simulink model "Interface_Model"  (R2017b)
settings: Solver=FixedStepDiscrete  StartTime=0.0  StopTime=inf  RelTol=1e-3  EnableMultiTasking=on
InitFcn:
  | modelSettings
undefined symbols (not defined in the file or in its folder): F, RadioSampleRate
libraries: gm_combinedTxRx_ExternalMode_lib x3
settings Model: SimulationMode=external  Creator=tcollins  LastModifiedBy=tcollins
settings SolverCC: PositivePriorityOrder=on
settings OptimizationCC: BlockReduction=off  ConditionallyExecuteInputs=off  PassReuseOutputArgsAs=Individual arguments  MaxStackSize=64
settings DebuggingCC: AlgebraicLoopMsg=error  SingleTaskRateTransMsg=error  ParameterTunabilityLossMsg=error
settings HardwareCC: ProdBitPerPointer=32  ProdBitPerSizeT=32  ProdBitPerPtrDiffT=32  ProdLargestAtomicInteger=Long  ProdLargestAtomicFloat=Double  ProdWordSize=32  ProdLongLongMode=on  ProdHWDeviceType=ARM Compatible->ARM Cortex  TargetLargestAtomicInteger=Long  TargetLargestAtomicFloat=Double  TargetIntDivRoundTo=Zero  TargetEndianess=LittleEndian  TargetHWDeviceType=ARM Compatible->ARM Cortex
settings SFSimCC: MATLABDynamicMemAlloc=off
settings RTWCC: SystemTargetFile=ert.tlc  HardwareBoard=Xilinx Zynq Based Radio Board Target  TemplateMakefile=ert_default_tmf  GenerateReport=on  Toolchain=Xilinx Software Development Kit (SDK)  IncludeHyperlinkInReport=on  LaunchReport=on  GenerateTraceInfo=on  GenerateTraceReport=on  GenerateTraceReportSl=on  GenerateTraceReportSf=on  GenerateTraceReportEml=on
settings CodeAppCC: ForceParamTrailComments=on  IgnoreCustomStorageClasses=off  OperatorAnnotations=on  SimulinkDataObjDesc=on  SFDataObjDesc=on  InsertBlockDesc=on

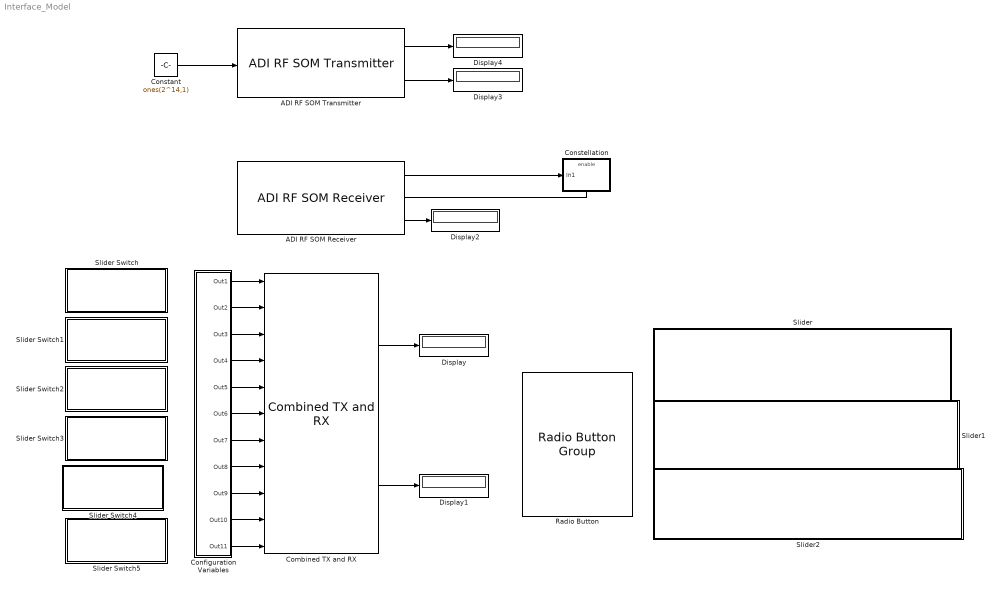
== system Interface_Model ==
  ADI RF SOM Receiver : gm_combinedTxRx_ExternalMode_lib/ADI RF SOM Receiver  IPAddress=192.168.3.2  CenterFrequencySource=Dialog  CenterFrequency=2400000000  GainSource=AGC Slow Attack  Gain=1  ChannelMapping=1  BasebandSampleRate=1e6  EnableBurstMode=off  NumFramesInBurst=20  OutputDataType=int16  SamplesPerFrame=2^14  LostSamplesOutputPort=on  RSSIOutputPort=off  DMATimeoutValue=1  blockMode=Codegen  SimulateUsing=Code generation  EnableQuadratureTracking=on  EnableRFDCTracking=on  EnableBasebandDCTracking=on  BypassUserLogic=off  ShowAdvancedProperties=on  ShowInternalProperties=off  subDeviceList=zynqReceiver  sdrExecutionMode=HW  dataUDPPort=-1  ctrlUDPPort=-1  SourceSelect=RF data  SourceConfiguration1=1023  FIRCoefficientSize=[ 128; 128 ]  FIRCoefficients=[ 55, -54, 42, -126, -123, -317, -399, -581, -646, -711, -634, -507, -263, -10, 255, 424, 492, 401, 201, -84, -352, -540, -566, -423, -126, 234, 562, 738, 701, 429, -5, -490, -866, -1007, -834, -372, 266, 891, 1301, 1334, 936, 178, -733, -1524, -1917, -1731, -944, 274, 1590, 2585, 2881, 2255, 741, -1344, -3435, -4850, -4942, -3285, 197, 5169, 10923, 16509, 20932, 23375, 23375, 20932, 16509, 10923, 5169, 197, -3285, -4942, -4850, -3435, -1344, 741, 2255, 2881, 2585, 1590, 274, -944, -1731, -1917, -1524, -733, 178, 936, 1334, 1301, 891, 266, -372, -834, -1007, -866, -490, -5, 429, 701, 738, 562, 234, -126, -423, -566, -540, -352, -84, 201, 401, 492, 424, 255, -10, -263, -507, -634, -711, -646, -581, -399, -317, -123, -126, 42, -54, 55; 190, -88, 329, -40, 239, -99, -24, -349, -377, -611, -573, -604, -395, -229, 66, 239, 394, 350, 227, -46, -300, -534, -593, -506, -221, 137, 512, 737, 765, 526, 103, -420, -852, -1069, -947, -512, 156, 841, 1341, 1450, 1100, 333, -638, -1531, -2028, -1922, -1152, 115, 1544, 2677, 3099, 2535, 997, -1205, -3479, -5095, -5345, -3750, -199, 4965, 11002, 16895, 21580, 24172, 24172, 21580, 16895, 11002, 4965, -199, -3750, -5345, -5095, -3479, -1205, 997, 2535, 3099, 2677, 1544, 115, -1152, -1922, -2028, -1531, -638, 333, 1100, 1450, 1341, 841, 156, -512, -947, -1069, -852, -420, 103, 526, 765, 737, 512, 137, -221, -506, -593, -534, -300, -46, 227, 350, 394, 239, 66, -229, -395, -604, -573, -611, -377, -349, -24, -99, 239, -40, 329, -88, 190 ]  FIRGain=[ 0; -12 ]  FIRDecimInterpFactor=[ 4; 4 ]  AnalogFilterCutoff=[ 3152524; 3161715 ]  FilterPathRates=[ 983040000, 122880000, 61440000, 30720000, 15360000, 3840000; 983040000, 122880000, 61440000, 30720000, 15360000, 3840000 ]  FilterDesignTypeForTx=DefaultFilterFromOther  FilterDesignTypeForRx=DefaultFilter  BISTLoopbackConfig=No Loopback  BISTPRBSMode=PRBS Disable  BISTToneMode=Tone Disable  BISTToneFrequency=F/32  BISTToneLevel=-6  BISTChannelMask=0  DataIsComplex=on
  ADI RF SOM Transmitter : gm_combinedTxRx_ExternalMode_lib/ADI RF SOM Transmitter  IPAddress=192.168.3.2  CenterFrequencySource=Dialog  CenterFrequency=2400000000  GainSource=Dialog  Gain=-10  ChannelMapping=1  BasebandSampleRate=1e6  EnableBurstMode=off  NumFramesInBurst=20  DMATimeoutValue=1  EnableTxPrimingMode=on  blockMode=Codegen  LostSamplesOutputPort=on  OverflowOutputPort=off  SimulateUsing=Code generation  DataSourceSelect=Host  DDSFrequency=[ 1000000, 1000000; 1000000, 1000000 ]  DDSPhase=[ 0, 0; 0, 0 ]  DDSScale=[ 250000, 250000; 250000, 250000 ]  BypassUserLogic=off  ShowAdvancedProperties=on  ShowInternalProperties=off  subDeviceList=zynqTransmitter  sdrExecutionMode=HW  dataUDPPort=-1  ctrlUDPPort=-1  FIRCoefficientSize=[ 128; 128 ]  FIRCoefficients=[ 55, -54, 42, -126, -123, -317, -399, -581, -646, -711, -634, -507, -263, -10, 255, 424, 492, 401, 201, -84, -352, -540, -566, -423, -126, 234, 562, 738, 701, 429, -5, -490, -866, -1007, -834, -372, 266, 891, 1301, 1334, 936, 178, -733, -1524, -1917, -1731, -944, 274, 1590, 2585, 2881, 2255, 741, -1344, -3435, -4850, -4942, -3285, 197, 5169, 10923, 16509, 20932, 23375, 23375, 20932, 16509, 10923, 5169, 197, -3285, -4942, -4850, -3435, -1344, 741, 2255, 2881, 2585, 1590, 274, -944, -1731, -1917, -1524, -733, 178, 936, 1334, 1301, 891, 266, -372, -834, -1007, -866, -490, -5, 429, 701, 738, 562, 234, -126, -423, -566, -540, -352, -84, 201, 401, 492, 424, 255, -10, -263, -507, -634, -711, -646, -581, -399, -317, -123, -126, 42, -54, 55; 190, -88, 329, -40, 239, -99, -24, -349, -377, -611, -573, -604, -395, -229, 66, 239, 394, 350, 227, -46, -300, -534, -593, -506, -221, 137, 512, 737, 765, 526, 103, -420, -852, -1069, -947, -512, 156, 841, 1341, 1450, 1100, 333, -638, -1531, -2028, -1922, -1152, 115, 1544, 2677, 3099, 2535, 997, -1205, -3479, -5095, -5345, -3750, -199, 4965, 11002, 16895, 21580, 24172, 24172, 21580, 16895, 11002, 4965, -199, -3750, -5345, -5095, -3479, -1205, 997, 2535, 3099, 2677, 1544, 115, -1152, -1922, -2028, -1531, -638, 333, 1100, 1450, 1341, 841, 156, -512, -947, -1069, -852, -420, 103, 526, 765, 737, 512, 137, -221, -506, -593, -534, -300, -46, 227, 350, 394, 239, 66, -229, -395, -604, -573, -611, -377, -349, -24, -99, 239, -40, 329, -88, 190 ]  FIRGain=[ 0; -12 ]  FIRDecimInterpFactor=[ 4; 4 ]  AnalogFilterCutoff=[ 3152524; 3161715 ]  FilterPathRates=[ 983040000, 122880000, 61440000, 30720000, 15360000, 3840000; 983040000, 122880000, 61440000, 30720000, 15360000, 3840000 ]  FilterDesignTypeForTx=DefaultFilter  FilterDesignTypeForRx=DefaultFilterFromOther
  Combined TX and RX : gm_combinedTxRx_ExternalMode_lib/Combined TX and RX
  Configuration Variables : Subsystem
  Constant : Constant  Value=ones(2^14,1)  SampleTime=-1
  Constellation : Subsystem
  Display{,1..4} (5 alike) : Display
  Radio Button : RadioButtonGroup  WebBlockId=323  ModelName=Interface_Model  LabelPosition=Top  ShowInitialText=on  SelectedLabel=After SRRC  ButtonGroupName=Constellation Data Source
      settings: Values={{'After SRRC', 'After Timing Recovery', 'After Frequency Recovery', 'After EQ'}, [1 2 3 4]}
  Slider : Subsystem  DialogController=hmiCreateDDGDialog  IsWebBlock=on  mask(MWDashboardBlock){webBlockId=d4feb81d-cb24-4eef-b536-d200a1891d41, webBlockType=slider, ShowInLibBrowser=on, ShowInitialText=on, HMISrcModelName=Interface_Model}
      mask prompts: webBlockId "WebBlock Id"; webBlockType "WebBlock Type"; HMISrcModelName "Source Model"
      mask help: SimulinkHMI:dialogs:SliderDialogDesc
      mask Help: helpview([docroot '/mapfiles/simulink.map'], 'hmi_slider')
      mask Display:
      | if strcmp(get_param(bdroot(gcb),'BlockDiagramType'), 'library')
      |     image([(matlabroot) '/toolbox/simulink/hmi/icons/Slider.png']);
      | end
  Slider Switch : Subsystem  DialogController=hmiCreateDDGDialog  IsWebBlock=on  mask(MWDashboardBlock){webBlockId=26219f1f-1109-40ca-a4af-2a8bc964a3a4, webBlockType=sliderswitch, ShowInLibBrowser=on, ShowInitialText=on, HMISrcModelName=Interface_Model}
      mask prompts: webBlockId "WebBlock Id"; webBlockType "WebBlock Type"; HMISrcModelName "Source Model"
      mask help: SimulinkHMI:dialogs:SwitchDialogDesc
      mask Help: helpview([docroot '/mapfiles/simulink.map'], 'hmi_slider_switch')
      mask Display:
      | if strcmp(get_param(bdroot(gcb),'BlockDiagramType'), 'library')
      |     image([(matlabroot) '/toolbox/simulink/hmi/icons/SliderSwitch.png']);
      | end
  Slider Switch1 : Subsystem  DialogController=hmiCreateDDGDialog  IsWebBlock=on  mask(MWDashboardBlock){webBlockId=1eddc475-4e28-4e7e-8fa4-3c106ebddf36, webBlockType=sliderswitch, ShowInLibBrowser=on, ShowInitialText=on, HMISrcModelName=Interface_Model}
      mask prompts: webBlockId "WebBlock Id"; webBlockType "WebBlock Type"; HMISrcModelName "Source Model"
      mask help: SimulinkHMI:dialogs:SwitchDialogDesc
      mask Help: helpview([docroot '/mapfiles/simulink.map'], 'hmi_slider_switch')
      mask Display:
      | if strcmp(get_param(bdroot(gcb),'BlockDiagramType'), 'library')
      |     image([(matlabroot) '/toolbox/simulink/hmi/icons/SliderSwitch.png']);
      | end
  Slider Switch2 : Subsystem  DialogController=hmiCreateDDGDialog  IsWebBlock=on  mask(MWDashboardBlock){webBlockId=eeafa1fd-631f-4ad5-a162-b269cb845515, webBlockType=sliderswitch, ShowInLibBrowser=on, ShowInitialText=on, HMISrcModelName=Interface_Model}
      mask prompts: webBlockId "WebBlock Id"; webBlockType "WebBlock Type"; HMISrcModelName "Source Model"
      mask help: SimulinkHMI:dialogs:SwitchDialogDesc
      mask Help: helpview([docroot '/mapfiles/simulink.map'], 'hmi_slider_switch')
      mask Display:
      | if strcmp(get_param(bdroot(gcb),'BlockDiagramType'), 'library')
      |     image([(matlabroot) '/toolbox/simulink/hmi/icons/SliderSwitch.png']);
      | end
  Slider Switch3 : Subsystem  DialogController=hmiCreateDDGDialog  IsWebBlock=on  mask(MWDashboardBlock){webBlockId=d26f103e-6633-4623-a5ec-df427e9233ad, webBlockType=sliderswitch, ShowInLibBrowser=on, ShowInitialText=on, HMISrcModelName=Interface_Model}
      mask prompts: webBlockId "WebBlock Id"; webBlockType "WebBlock Type"; HMISrcModelName "Source Model"
      mask help: SimulinkHMI:dialogs:SwitchDialogDesc
      mask Help: helpview([docroot '/mapfiles/simulink.map'], 'hmi_slider_switch')
      mask Display:
      | if strcmp(get_param(bdroot(gcb),'BlockDiagramType'), 'library')
      |     image([(matlabroot) '/toolbox/simulink/hmi/icons/SliderSwitch.png']);
      | end
  Slider Switch4 : Subsystem  DialogController=hmiCreateDDGDialog  IsWebBlock=on  mask(MWDashboardBlock){webBlockId=ba810177-532f-4366-b8e7-2a0e810ca864, webBlockType=sliderswitch, ShowInLibBrowser=on, ShowInitialText=on, HMISrcModelName=Interface_Model}
      mask prompts: webBlockId "WebBlock Id"; webBlockType "WebBlock Type"; HMISrcModelName "Source Model"
      mask help: SimulinkHMI:dialogs:SwitchDialogDesc
      mask Help: helpview([docroot '/mapfiles/simulink.map'], 'hmi_slider_switch')
      mask Display:
      | if strcmp(get_param(bdroot(gcb),'BlockDiagramType'), 'library')
      |     image([(matlabroot) '/toolbox/simulink/hmi/icons/SliderSwitch.png']);
      | end
  Slider Switch5 : Subsystem  DialogController=hmiCreateDDGDialog  IsWebBlock=on  mask(MWDashboardBlock){webBlockId=216110c8-cc91-453d-9952-97baaa76ee3d, webBlockType=sliderswitch, ShowInLibBrowser=on, ShowInitialText=on, HMISrcModelName=Interface_Model}
      mask prompts: webBlockId "WebBlock Id"; webBlockType "WebBlock Type"; HMISrcModelName "Source Model"
      mask help: SimulinkHMI:dialogs:SwitchDialogDesc
      mask Help: helpview([docroot '/mapfiles/simulink.map'], 'hmi_slider_switch')
      mask Display:
      | if strcmp(get_param(bdroot(gcb),'BlockDiagramType'), 'library')
      |     image([(matlabroot) '/toolbox/simulink/hmi/icons/SliderSwitch.png']);
      | end
  Slider1 : Subsystem  DialogController=hmiCreateDDGDialog  IsWebBlock=on  mask(MWDashboardBlock){webBlockId=ada10824-bcdc-457e-86db-13bcc653ecfd, webBlockType=slider, ShowInLibBrowser=on, ShowInitialText=on, HMISrcModelName=Interface_Model}
      mask prompts: webBlockId "WebBlock Id"; webBlockType "WebBlock Type"; HMISrcModelName "Source Model"
      mask help: SimulinkHMI:dialogs:SliderDialogDesc
      mask Help: helpview([docroot '/mapfiles/simulink.map'], 'hmi_slider')
      mask Display:
      | if strcmp(get_param(bdroot(gcb),'BlockDiagramType'), 'library')
      |     image([(matlabroot) '/toolbox/simulink/hmi/icons/Slider.png']);
      | end
  Slider2 : Subsystem  DialogController=hmiCreateDDGDialog  IsWebBlock=on  mask(MWDashboardBlock){webBlockId=948c7412-cd60-4ac0-9221-40aef6caa45a, webBlockType=slider, ShowInLibBrowser=on, ShowInitialText=on, HMISrcModelName=Interface_Model}
      mask prompts: webBlockId "WebBlock Id"; webBlockType "WebBlock Type"; HMISrcModelName "Source Model"
      mask help: SimulinkHMI:dialogs:SliderDialogDesc
      mask Help: helpview([docroot '/mapfiles/simulink.map'], 'hmi_slider')
      mask Display:
      | if strcmp(get_param(bdroot(gcb),'BlockDiagramType'), 'library')
      |     image([(matlabroot) '/toolbox/simulink/hmi/icons/Slider.png']);
      | end
  wires:
  Configuration Variables/11(Out11) -> Combined TX and RX/11
  Configuration Variables/10(Out10) -> Combined TX and RX/10
  Configuration Variables/9(Out9) -> Combined TX and RX/9
  Configuration Variables/8(Out8) -> Combined TX and RX/8
  Configuration Variables/7(Out7) -> Combined TX and RX/7
  Configuration Variables/6(Out6) -> Combined TX and RX/6
  Configuration Variables/5(Out5) -> Combined TX and RX/5
  Configuration Variables/4(Out4) -> Combined TX and RX/4
  Configuration Variables/3(Out3) -> Combined TX and RX/3
  Configuration Variables/2(Out2) -> Combined TX and RX/2
  Configuration Variables/1(Out1) -> Combined TX and RX/1
  Combined TX and RX/1 -> Display/1
  Combined TX and RX/2 -> Display1/1
  ADI RF SOM Receiver/3 -> Display2/1
  ADI RF SOM Receiver/2 -> Constellation/Enable
  ADI RF SOM Receiver/1 -> Constellation/1(In1)
  Constant/1 -> ADI RF SOM Transmitter/1
  ADI RF SOM Transmitter/2 -> Display3/1
  ADI RF SOM Transmitter/1 -> Display4/1

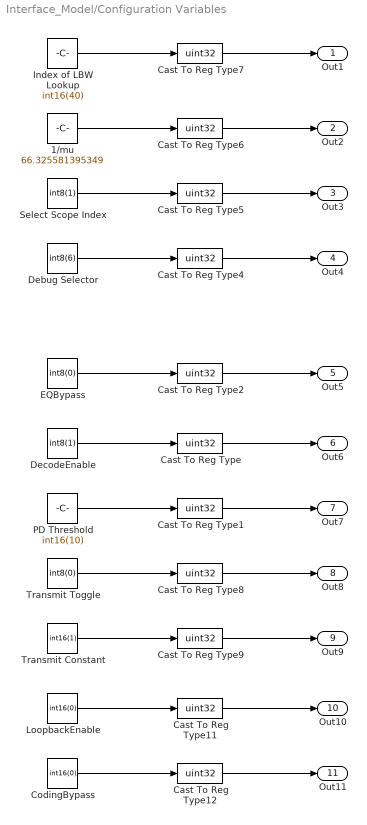
== system Interface_Model/Configuration Variables ==
  1/mu : Constant  Value=66.325581395349  OutDataTypeStr=int16  SampleTime=-1
  Cast To Reg Type{,1..2,4..9,11..12} (11 alike) : DataTypeConversion  OutDataTypeStr=uint32
  CodingBypass : Constant  Value=int16(0)  SampleTime=1/RadioSampleRate
  Debug Selector : Constant  Value=int8(6)  SampleTime=1/RadioSampleRate
  DecodeEnable : Constant  Value=int8(1)  SampleTime=1/RadioSampleRate
  EQBypass : Constant  Value=int8(0)  SampleTime=1/RadioSampleRate
  Index of LBW Lookup : Constant  Value=int16(40)  SampleTime=1/RadioSampleRate
  LoopbackEnable : Constant  Value=int16(0)  SampleTime=1/RadioSampleRate
  PD Threshold : Constant  Value=int16(10)  SampleTime=1/RadioSampleRate
  Select Scope Index : Constant  Value=int8(1)  SampleTime=1/RadioSampleRate
  Transmit Constant : Constant  Value=int16(1)  SampleTime=1/RadioSampleRate
  Transmit Toggle : Constant  Value=int8(0)  SampleTime=1/RadioSampleRate
  Out1 : Outport
  Out2 : Outport  Port=2
  Out3 : Outport  Port=3
  Out4 : Outport  Port=4
  Out5 : Outport  Port=5
  Out6 : Outport  Port=6
  Out7 : Outport  Port=7
  Out8 : Outport  Port=8
  Out9 : Outport  Port=9
  Out10 : Outport  Port=10
  Out11 : Outport  Port=11
  wires:
  1/mu/1 -> Cast To Reg Type6/1
  Index of LBW Lookup/1 -> Cast To Reg Type7/1
  Select Scope Index/1 -> Cast To Reg Type5/1
  Debug Selector/1 -> Cast To Reg Type4/1
  EQBypass/1 -> Cast To Reg Type2/1
  DecodeEnable/1 -> Cast To Reg Type/1
  PD Threshold/1 -> Cast To Reg Type1/1
  Cast To Reg Type1/1 -> Out7/1
  Cast To Reg Type/1 -> Out6/1
  Cast To Reg Type2/1 -> Out5/1
  Cast To Reg Type4/1 -> Out4/1
  Cast To Reg Type5/1 -> Out3/1
  Cast To Reg Type6/1 -> Out2/1
  Cast To Reg Type7/1 -> Out1/1
  Transmit Toggle/1 -> Cast To Reg Type8/1
  Transmit Constant/1 -> Cast To Reg Type9/1
  Cast To Reg Type9/1 -> Out9/1
  Cast To Reg Type8/1 -> Out8/1
  LoopbackEnable/1 -> Cast To Reg Type11/1
  Cast To Reg Type11/1 -> Out10/1
  CodingBypass/1 -> Cast To Reg Type12/1
  Cast To Reg Type12/1 -> Out11/1

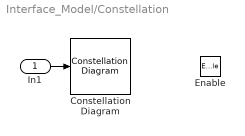
== system Interface_Model/Constellation ==
  In1 : Inport
  Enable : EnablePort
  Constellation Diagram : ConstellationDiagram
  wires:
  In1/1 -> Constellation Diagram/1

== system Interface_Model/Slider ==

== system Interface_Model/Slider Switch ==

== system Interface_Model/Slider Switch1 ==

== system Interface_Model/Slider Switch2 ==

== system Interface_Model/Slider Switch3 ==

== system Interface_Model/Slider Switch4 ==

== system Interface_Model/Slider Switch5 ==

== system Interface_Model/Slider1 ==

== system Interface_Model/Slider2 ==
